simulink model "HANcoder_E407_GTSync_v5"  (R2018b)
settings: Solver=FixedStepDiscrete  StartTime=0.0  StopTime=1  FixedStep=0.01  RelTol=1e-3
PreLoadFcn:
  | librarySetup
  | eval([bdroot,'_startup']) %Calling [modelName]_startup.m
values from neighbouring files (symbols this model uses):
  basic_cycle_duration = TM_Reset_Board + COMP_duration    (= 170)    [HANcoder_E407_GTSync_v5_startup.m]
  comm_delay_estimation1 = round(comm_delay_measured*hardware_granularity/frequency_IRQ)    [HANcoder_E407_GTSync_v5_startup.m]
  comm_delay_estimation2 = round(comm_delay_measured*hardware_granularity/frequency_IRQ)    [HANcoder_E407_GTSync_v5_startup.m]
  COMM_Period = 25    [HANcoder_E407_GTSync_v5_startup.m]
  COMM_Phase1 = floor(COMM_Period/5)    [HANcoder_E407_GTSync_v5_startup.m]
  COMM_Phase2 = floor(4*COMM_Period/5)    [HANcoder_E407_GTSync_v5_startup.m]
  frequency_IRQ = 100    [HANcoder_E407_GTSync_v5_startup.m]
  HANtuneOverride = Simulink.Parameter    [HANcoder_E407_GTSync_v5_startup.m]
  idle_time_init = basic_cycle_duration*matrix_rows    (= 340)    [HANcoder_E407_GTSync_v5_startup.m]
  LED_ticks_toggle = 10000    [HANcoder_E407_GTSync_v5_startup.m]
  Master_Role = 1    [HANcoder_E407_GTSync_v5_startup.m]
  matrix_rows = 2    [HANcoder_E407_GTSync_v5_startup.m]
  MEX_Flag = 0    [HANcoder_E407_GTSync_v5_startup.m]
  Slave_Role = 2    [HANcoder_E407_GTSync_v5_startup.m]
  Sync_ID = 1    [HANcoder_E407_GTSync_v5_startup.m]
  TM_Check_Sync = TM_COMM_Sync   + COMM_duration    (= 30)    [HANcoder_E407_GTSync_v5_startup.m]
  TM_Check_TOuts = TM_Count_Vote3 + COMP_duration    (= 150)    [HANcoder_E407_GTSync_v5_startup.m]
  TM_Check_Vote1 = TM_COMM_Vote1  + COMM_duration    (= 70)    [HANcoder_E407_GTSync_v5_startup.m]
  TM_Check_Vote2 = TM_COMM_Vote2  + COMM_duration    (= 105)    [HANcoder_E407_GTSync_v5_startup.m]
  TM_Check_Vote3 = TM_COMM_Vote3  + COMM_duration    (= 140)    [HANcoder_E407_GTSync_v5_startup.m]
  TM_COMM_Sync = basic_cycle_start    (= 5)    [HANcoder_E407_GTSync_v5_startup.m]
  TM_COMM_Vote1 = TM_Vote_Dec    + COMP_duration    (= 45)    [HANcoder_E407_GTSync_v5_startup.m]
  TM_COMM_Vote2 = TM_Count_Vote1 + COMP_duration    (= 80)    [HANcoder_E407_GTSync_v5_startup.m]
  TM_COMM_Vote3 = TM_Count_Vote2 + COMP_duration    (= 115)    [HANcoder_E407_GTSync_v5_startup.m]
  TM_Count_Vote1 = TM_Check_Vote1 + COMP_duration    (= 75)    [HANcoder_E407_GTSync_v5_startup.m]
  TM_Count_Vote2 = TM_Check_Vote2 + COMP_duration    (= 110)    [HANcoder_E407_GTSync_v5_startup.m]
  TM_Count_Vote3 = TM_Check_Vote3 + COMP_duration    (= 145)    [HANcoder_E407_GTSync_v5_startup.m]
  TM_New_Master = TM_Check_TOuts + COMP_duration    (= 155)    [HANcoder_E407_GTSync_v5_startup.m]
  TM_Reset_Board = TM_Reset_Var   + COMP_duration    (= 165)    [HANcoder_E407_GTSync_v5_startup.m]
  TM_Reset_Var = TM_New_Master  + COMP_duration    (= 160)    [HANcoder_E407_GTSync_v5_startup.m]
  TM_Update_LT = TM_Check_Sync  + COMP_duration    (= 35)    [HANcoder_E407_GTSync_v5_startup.m]
  TM_Vote_Dec = TM_Update_LT   + COMP_duration    (= 40)    [HANcoder_E407_GTSync_v5_startup.m]
  Toggle_Flag = 1    [HANcoder_E407_GTSync_v5_startup.m]
  Vote1_ID = 12    [HANcoder_E407_GTSync_v5_startup.m]
  Vote2_ID = 22    [HANcoder_E407_GTSync_v5_startup.m]
  Vote3_ID = 32    [HANcoder_E407_GTSync_v5_startup.m]
undefined symbols (not defined in the file or in its folder): A0, A1, A2, A3, CON2
libraries: HANcoder_STM32_Target x25, hdlsllib x21, simulink x3, simulink_extras x1
(part 5 of 7)

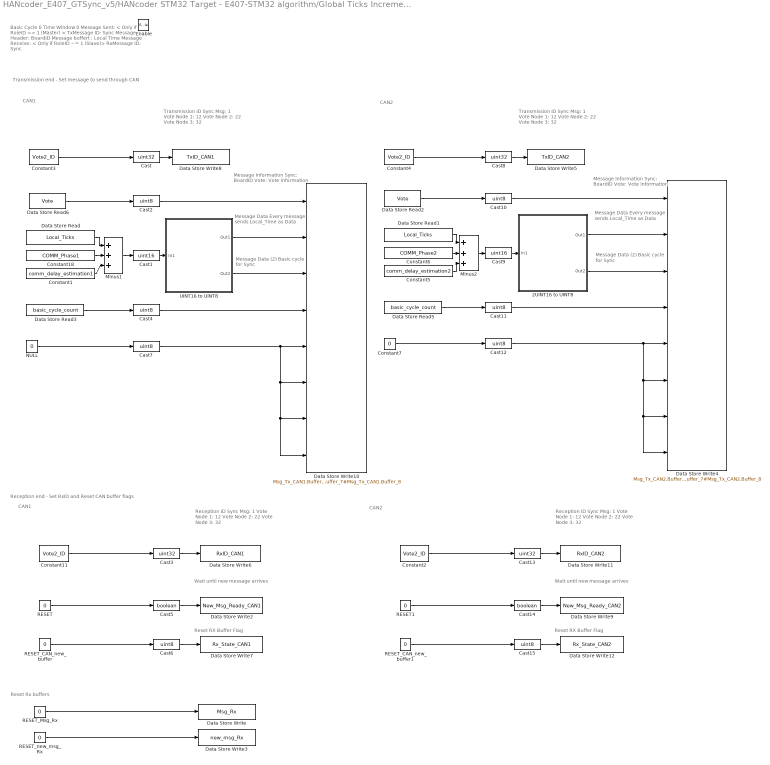
== system HANcoder_E407_GTSync_v5/HANcoder STM32 Target - E407-STM32 algorithm/Global Ticks Increment/CAN Management/Matrix Cycle Manager/COMM Task - Vote2/Vote 2 ==
  note: CAN2
  note: CAN1
  note: Transmission end - Set message to send through CAN
  note: CAN2
  note: CAN1
  note: Reception end - Set RxID and Reset CAN buffer flags
  note: Reset Rx buffers
  note: Wait until new message
      | arrives
  note: Message Data (2)
      |    Basic cycle for Sync
  note: Basic Cycle 0
      | Time Window 0
      | Message Sent: < Only if RoleID == 1 (Master) >
      | 	TxMessage ID: Sync
      | 	Message Header: BoardID
      | 	Message buffert : Local Time
      | Message Receive: < Only if RoleID ~= 1 (Slave)>
      | 	RxMessage ID: Sync
  note: Message Data
      |    Every message sends
      |    Local_Time as Data
  note: Transmission ID
      |    Sync Msg: 1
      |    Vote Node 1: 12
      |    Vote Node 2: 22
      |    Vote Node 3: 32
  note: Message Information
      |    Sync: BoardID
      |    Vote: Vote information
  note: Reception ID
      |    Sync Msg: 1
      |    Vote Node 1: 12
      |    Vote Node 2: 22
      |    Vote Node 3: 32
  note: Reset RX Buffer Flag
  note: Message Data (2)
      |    Basic cycle for Sync
  note: Message Data
      |    Every message sends
      |    Local_Time as Data
  note: Transmission ID
      |    Sync Msg: 1
      |    Vote Node 1: 12
      |    Vote Node 2: 22
      |    Vote Node 3: 32
  note: Message Information
      |    Sync: BoardID
      |    Vote: Vote information
  note: Wait until new message
      | arrives
  note: Reception ID
      |    Sync Msg: 1
      |    Vote Node 1: 12
      |    Vote Node 2: 22
      |    Vote Node 3: 32
  note: Reset RX Buffer Flag
  Enable : EnablePort
  2UINT16 to UINT8 : Subsystem
  Cast{,3,8,13} (4 alike) : DataTypeConversion  OutDataTypeStr=uint32
  Cast1 : DataTypeConversion  OutDataTypeStr=uint16
  Cast{2,4,6..7,10..12,15} (8 alike) : DataTypeConversion  OutDataTypeStr=uint8
  Cast14 : DataTypeConversion  OutDataTypeStr=boolean
  Cast5 : DataTypeConversion  OutDataTypeStr=boolean
  Cast9 : DataTypeConversion  OutDataTypeStr=uint16
  Constant1 : Constant  Value=comm_delay_estimation1
  Constant{2..4,11} (4 alike) : Constant  Value=Vote2_ID
  Constant18 : Constant  Value=COMM_Phase1
  Constant5 : Constant  Value=comm_delay_estimation2
  Constant6 : Constant  Value=COMM_Phase2
  Constant7 : Constant  Value=0  OutDataTypeStr=uint8
  Data Store Read : DataStoreRead  DataStoreName=Local_Ticks
  Data Store Read1 : DataStoreRead  DataStoreName=Local_Ticks
  Data Store Read2 : DataStoreRead  DataStoreName=Vote
  Data Store Read3 : DataStoreRead  DataStoreName=basic_cycle_count
  Data Store Read5 : DataStoreRead  DataStoreName=basic_cycle_count
  Data Store Read6 : DataStoreRead  DataStoreName=Vote
  Data Store Write : DataStoreWrite  DataStoreName=Msg_Rx
  Data Store Write10 : DataStoreWrite  DataStoreName=Msg_Tx_CAN1  DataStoreElements=Msg_Tx_CAN1.Buffer_1#Msg_Tx_CAN1.Buffer_2#Msg_Tx_CAN1.Buffer_3#Msg_Tx_CAN1.Buffer_4#Msg_Tx_CAN1.Buffer_5#Msg_Tx_CAN1.Buffer_6#Msg_Tx_CAN1.Buffer_7#Msg_Tx_CAN1.Buffer_8
  Data Store Write11 : DataStoreWrite  DataStoreName=RxID_CAN2
  Data Store Write12 : DataStoreWrite  DataStoreName=Rx_State_CAN2
  Data Store Write2 : DataStoreWrite  DataStoreName=New_Msg_Ready_CAN1
  Data Store Write3 : DataStoreWrite  DataStoreName=new_msg_Rx
  Data Store Write4 : DataStoreWrite  DataStoreName=Msg_Tx_CAN2  DataStoreElements=Msg_Tx_CAN2.Buffer_1#Msg_Tx_CAN2.Buffer_2#Msg_Tx_CAN2.Buffer_3#Msg_Tx_CAN2.Buffer_4#Msg_Tx_CAN2.Buffer_5#Msg_Tx_CAN2.Buffer_6#Msg_Tx_CAN2.Buffer_7#Msg_Tx_CAN2.Buffer_8
  Data Store Write5 : DataStoreWrite  DataStoreName=TxID_CAN2
  Data Store Write6 : DataStoreWrite  DataStoreName=RxID_CAN1
  Data Store Write7 : DataStoreWrite  DataStoreName=Rx_State_CAN1
  Data Store Write8 : DataStoreWrite  DataStoreName=TxID_CAN1
  Data Store Write9 : DataStoreWrite  DataStoreName=New_Msg_Ready_CAN2
  Minus1 : Sum  Inputs=+++
  Minus2 : Sum  Inputs=+++
  NULL : Constant  Value=0  OutDataTypeStr=uint8
  RESET : Constant  Value=0
  RESET1 : Constant  Value=0
  RESET_CAN_new_buffer : Constant  Value=0
  RESET_CAN_new_buffer1 : Constant  Value=0
  RESET_Msg_Rx : Constant  Value=0  OutDataTypeStr=Bus: demux_msg_buffer_type
  RESET_new_msg_Rx : Constant  Value=0  OutDataTypeStr=boolean
  UINT16 to UINT8 : Subsystem
  wires:
  Constant18/1 -> Minus1/2
  Minus1/1 -> Cast1/1
  Cast/1 -> Data Store Write8/1
  Data Store Read/1 -> Minus1/1
  Constant3/1 -> Cast/1
  Cast3/1 -> Data Store Write6/1
  Constant11/1 -> Cast3/1
  Cast2/1 -> Data Store Write10/1
  Cast4/1 -> Data Store Write10/4
  Data Store Read3/1 -> Cast4/1
  Data Store Read6/1 -> Cast2/1
  RESET/1 -> Cast5/1
  Cast5/1 -> Data Store Write2/1
  RESET_Msg_Rx/1 -> Data Store Write/1
  RESET_new_msg_Rx/1 -> Data Store Write3/1
  RESET_CAN_new_buffer/1 -> Cast6/1
  Cast6/1 -> Data Store Write7/1
  Constant1/1 -> Minus1/3
  Cast1/1 -> UINT16 to UINT8/1(In1)
  UINT16 to UINT8/2(Out2) -> Data Store Write10/3
  UINT16 to UINT8/1(Out1) -> Data Store Write10/2
  Cast7/1 -> Data Store Write10/8, Data Store Write10/7, Data Store Write10/6, Data Store Write10/5
  NULL/1 -> Cast7/1
  Constant7/1 -> Cast12/1
  Cast12/1 -> Data Store Write4/8, Data Store Write4/7, Data Store Write4/6, Data Store Write4/5
  2UINT16 to UINT8/1(Out1) -> Data Store Write4/2
  2UINT16 to UINT8/2(Out2) -> Data Store Write4/3
  Cast9/1 -> 2UINT16 to UINT8/1(In1)
  Constant5/1 -> Minus2/3
  Data Store Read2/1 -> Cast10/1
  Data Store Read5/1 -> Cast11/1
  Cast11/1 -> Data Store Write4/4
  Cast10/1 -> Data Store Write4/1
  Constant4/1 -> Cast8/1
  Data Store Read1/1 -> Minus2/1
  Cast8/1 -> Data Store Write5/1
  Minus2/1 -> Cast9/1
  Constant6/1 -> Minus2/2
  Cast15/1 -> Data Store Write12/1
  RESET_CAN_new_buffer1/1 -> Cast15/1
  Cast14/1 -> Data Store Write9/1
  RESET1/1 -> Cast14/1
  Constant2/1 -> Cast13/1
  Cast13/1 -> Data Store Write11/1

== system HANcoder_E407_GTSync_v5/HANcoder STM32 Target - E407-STM32 algorithm/Global Ticks Increment/CAN Management/Matrix Cycle Manager/COMM Task - Vote3/Vote 3 ==
  note: CAN2
  note: CAN1
  note: Transmission end - Set message to send through CAN
  note: CAN2
  note: CAN1
  note: Reception end - Set RxID and Reset CAN buffer flags
  note: Reset Rx buffers
  note: Wait until new message
      | arrives
  note: Message Data (2)
      |    Basic cycle for Sync
  note: Basic Cycle 0
      | Time Window 0
      | Message Sent: < Only if RoleID == 1 (Master) >
      | 	TxMessage ID: Sync
      | 	Message Header: BoardID
      | 	Message buffert : Local Time
      | Message Receive: < Only if RoleID ~= 1 (Slave)>
      | 	RxMessage ID: Sync
  note: Message Data
      |    Every message sends
      |    Local_Time as Data
  note: Transmission ID
      |    Sync Msg: 1
      |    Vote Node 1: 12
      |    Vote Node 2: 22
      |    Vote Node 3: 32
  note: Message Information
      |    Sync: BoardID
      |    Vote: Vote information
  note: Reception ID
      |    Sync Msg: 1
      |    Vote Node 1: 12
      |    Vote Node 2: 22
      |    Vote Node 3: 32
  note: Reset RX Buffer Flag
  note: Message Data (2)
      |    Basic cycle for Sync
  note: Message Data
      |    Every message sends
      |    Local_Time as Data
  note: Transmission ID
      |    Sync Msg: 1
      |    Vote Node 1: 12
      |    Vote Node 2: 22
      |    Vote Node 3: 32
  note: Message Information
      |    Sync: BoardID
      |    Vote: Vote information
  note: Wait until new message
      | arrives
  note: Reception ID
      |    Sync Msg: 1
      |    Vote Node 1: 12
      |    Vote Node 2: 22
      |    Vote Node 3: 32
  note: Reset RX Buffer Flag
  Enable : EnablePort
  2UINT16 to UINT8 : Subsystem
  Cast{,3,8,13} (4 alike) : DataTypeConversion  OutDataTypeStr=uint32
  Cast1 : DataTypeConversion  OutDataTypeStr=uint16
  Cast{2,4,6..7,10..12,15} (8 alike) : DataTypeConversion  OutDataTypeStr=uint8
  Cast14 : DataTypeConversion  OutDataTypeStr=boolean
  Cast5 : DataTypeConversion  OutDataTypeStr=boolean
  Cast9 : DataTypeConversion  OutDataTypeStr=uint16
  Constant1 : Constant  Value=comm_delay_estimation1
  Constant{2..4,11} (4 alike) : Constant  Value=Vote3_ID
  Constant18 : Constant  Value=COMM_Phase1
  Constant5 : Constant  Value=comm_delay_estimation2
  Constant6 : Constant  Value=COMM_Phase2
  Constant7 : Constant  Value=0  OutDataTypeStr=uint8
  Data Store Read : DataStoreRead  DataStoreName=Local_Ticks
  Data Store Read1 : DataStoreRead  DataStoreName=Local_Ticks
  Data Store Read2 : DataStoreRead  DataStoreName=Vote
  Data Store Read3 : DataStoreRead  DataStoreName=basic_cycle_count
  Data Store Read5 : DataStoreRead  DataStoreName=basic_cycle_count
  Data Store Read6 : DataStoreRead  DataStoreName=Vote
  Data Store Write : DataStoreWrite  DataStoreName=Msg_Rx
  Data Store Write10 : DataStoreWrite  DataStoreName=Msg_Tx_CAN1  DataStoreElements=Msg_Tx_CAN1.Buffer_1#Msg_Tx_CAN1.Buffer_2#Msg_Tx_CAN1.Buffer_3#Msg_Tx_CAN1.Buffer_4#Msg_Tx_CAN1.Buffer_5#Msg_Tx_CAN1.Buffer_6#Msg_Tx_CAN1.Buffer_7#Msg_Tx_CAN1.Buffer_8
  Data Store Write11 : DataStoreWrite  DataStoreName=RxID_CAN2
  Data Store Write12 : DataStoreWrite  DataStoreName=Rx_State_CAN2
  Data Store Write2 : DataStoreWrite  DataStoreName=New_Msg_Ready_CAN1
  Data Store Write3 : DataStoreWrite  DataStoreName=new_msg_Rx
  Data Store Write4 : DataStoreWrite  DataStoreName=Msg_Tx_CAN2  DataStoreElements=Msg_Tx_CAN2.Buffer_1#Msg_Tx_CAN2.Buffer_2#Msg_Tx_CAN2.Buffer_3#Msg_Tx_CAN2.Buffer_4#Msg_Tx_CAN2.Buffer_5#Msg_Tx_CAN2.Buffer_6#Msg_Tx_CAN2.Buffer_7#Msg_Tx_CAN2.Buffer_8
  Data Store Write5 : DataStoreWrite  DataStoreName=TxID_CAN2
  Data Store Write6 : DataStoreWrite  DataStoreName=RxID_CAN1
  Data Store Write7 : DataStoreWrite  DataStoreName=Rx_State_CAN1
  Data Store Write8 : DataStoreWrite  DataStoreName=TxID_CAN1
  Data Store Write9 : DataStoreWrite  DataStoreName=New_Msg_Ready_CAN2
  Minus1 : Sum  Inputs=+++
  Minus2 : Sum  Inputs=+++
  NULL : Constant  Value=0  OutDataTypeStr=uint8
  RESET : Constant  Value=0
  RESET1 : Constant  Value=0
  RESET_CAN_new_buffer : Constant  Value=0
  RESET_CAN_new_buffer1 : Constant  Value=0
  RESET_Msg_Rx : Constant  Value=0  OutDataTypeStr=Bus: demux_msg_buffer_type
  RESET_new_msg_Rx : Constant  Value=0  OutDataTypeStr=boolean
  UINT16 to UINT8 : Subsystem
  wires:
  Constant18/1 -> Minus1/2
  Minus1/1 -> Cast1/1
  Cast/1 -> Data Store Write8/1
  Data Store Read/1 -> Minus1/1
  Constant3/1 -> Cast/1
  Cast3/1 -> Data Store Write6/1
  Constant11/1 -> Cast3/1
  Cast2/1 -> Data Store Write10/1
  Cast4/1 -> Data Store Write10/4
  Data Store Read3/1 -> Cast4/1
  Data Store Read6/1 -> Cast2/1
  RESET/1 -> Cast5/1
  Cast5/1 -> Data Store Write2/1
  RESET_Msg_Rx/1 -> Data Store Write/1
  RESET_new_msg_Rx/1 -> Data Store Write3/1
  RESET_CAN_new_buffer/1 -> Cast6/1
  Cast6/1 -> Data Store Write7/1
  Constant1/1 -> Minus1/3
  Cast1/1 -> UINT16 to UINT8/1(In1)
  UINT16 to UINT8/2(Out2) -> Data Store Write10/3
  UINT16 to UINT8/1(Out1) -> Data Store Write10/2
  Cast7/1 -> Data Store Write10/8, Data Store Write10/7, Data Store Write10/6, Data Store Write10/5
  NULL/1 -> Cast7/1
  Constant7/1 -> Cast12/1
  Cast12/1 -> Data Store Write4/8, Data Store Write4/7, Data Store Write4/6, Data Store Write4/5
  2UINT16 to UINT8/1(Out1) -> Data Store Write4/2
  2UINT16 to UINT8/2(Out2) -> Data Store Write4/3
  Cast9/1 -> 2UINT16 to UINT8/1(In1)
  Constant5/1 -> Minus2/3
  Data Store Read2/1 -> Cast10/1
  Data Store Read5/1 -> Cast11/1
  Cast11/1 -> Data Store Write4/4
  Cast10/1 -> Data Store Write4/1
  Constant4/1 -> Cast8/1
  Data Store Read1/1 -> Minus2/1
  Cast8/1 -> Data Store Write5/1
  Minus2/1 -> Cast9/1
  Constant6/1 -> Minus2/2
  Cast15/1 -> Data Store Write12/1
  RESET_CAN_new_buffer1/1 -> Cast15/1
  Cast14/1 -> Data Store Write9/1
  RESET1/1 -> Cast14/1
  Constant2/1 -> Cast13/1
  Cast13/1 -> Data Store Write11/1

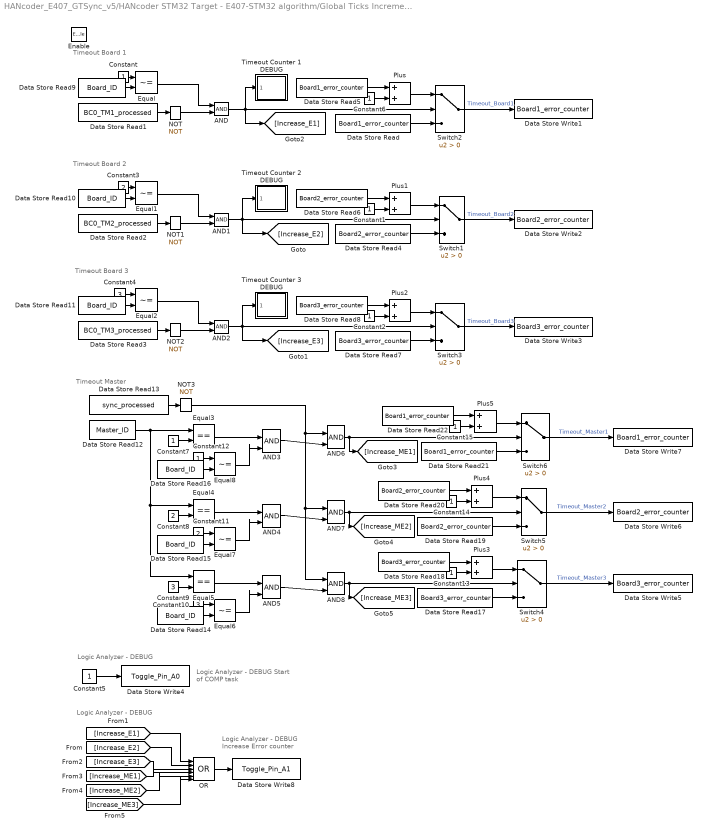
== system HANcoder_E407_GTSync_v5/HANcoder STM32 Target - E407-STM32 algorithm/Global Ticks Increment/CAN Management/Matrix Cycle Manager/COMP Task - Check Timeouts/Timeout and Board error counter ==
  note: Logic Analyzer - DEBUG
  note: Timeout Master
  note: Timeout Board 2
  note: Timeout Board 3
  note: Timeout Board 1
  note: Logic Analyzer - DEBUG
      | Start of COMP task
  note: Logic Analyzer - DEBUG
  note: Logic Analyzer - DEBUG
      | Increase Error counter
  Enable : EnablePort  PropagateVarSize=During execution
  AND{,1..8} (9 alike) : Logic  IconShape=distinctive  AllPortsSameDT=off  OutDataTypeStr=boolean
  Constant{,1..2,6..7,12..15} (9 alike) : Constant
  Constant10 : Constant  Value=3
  Constant11 : Constant  Value=2
  Constant3 : Constant  Value=2
  Constant4 : Constant  Value=3
  Constant5 : Constant  OutDataTypeStr=boolean
  Constant8 : Constant  Value=2
  Constant9 : Constant  Value=3
  Data Store Read{,5,21..22} (4 alike) : DataStoreRead  DataStoreName=Board1_error_counter
  Data Store Read1 : DataStoreRead  DataStoreName=BC0_TM1_processed
  Data Store Read{9..11,14..16} (6 alike) : DataStoreRead  DataStoreName=Board_ID
  Data Store Read12 : DataStoreRead  DataStoreName=Master_ID
  Data Store Read13 : DataStoreRead  DataStoreName=sync_processed
  Data Store Read{7..8,17..18} (4 alike) : DataStoreRead  DataStoreName=Board3_error_counter
  Data Store Read{4,6,19..20} (4 alike) : DataStoreRead  DataStoreName=Board2_error_counter
  Data Store Read2 : DataStoreRead  DataStoreName=BC0_TM2_processed
  Data Store Read3 : DataStoreRead  DataStoreName=BC0_TM3_processed
  Data Store Write1 : DataStoreWrite  DataStoreName=Board1_error_counter
  Data Store Write2 : DataStoreWrite  DataStoreName=Board2_error_counter
  Data Store Write3 : DataStoreWrite  DataStoreName=Board3_error_counter
  Data Store Write4 : DataStoreWrite  DataStoreName=Toggle_Pin_A0
  Data Store Write5 : DataStoreWrite  DataStoreName=Board3_error_counter
  Data Store Write6 : DataStoreWrite  DataStoreName=Board2_error_counter
  Data Store Write7 : DataStoreWrite  DataStoreName=Board1_error_counter
  Data Store Write8 : DataStoreWrite  DataStoreName=Toggle_Pin_A1
  Equal{,1..2,6..8} (6 alike) : RelationalOperator  Operator=~=  OutDataTypeStr=boolean  RndMeth=Simplest
  Equal3 : RelationalOperator  Operator===  OutDataTypeStr=boolean  RndMeth=Simplest
  Equal4 : RelationalOperator  Operator===  OutDataTypeStr=boolean  RndMeth=Simplest
  Equal5 : RelationalOperator  Operator===  OutDataTypeStr=boolean  RndMeth=Simplest
  NOT{,1..3} (4 alike) : Logic  Operator=NOT  IconShape=distinctive  AllPortsSameDT=off  OutDataTypeStr=boolean
  OR : Logic  Operator=OR  Inputs=6  IconShape=distinctive  AllPortsSameDT=off  OutDataTypeStr=boolean
  Plus{,1..5} (6 alike) : Sum
  Switch{1..6} (6 alike) : Switch  Criteria=u2 > Threshold
  Timeout Counter 1 DEBUG : Subsystem
  Timeout Counter 2 DEBUG : Subsystem
  Timeout Counter 3 DEBUG : Subsystem
  wires:
  Constant6/1 -> Plus/2
  Plus/1 -> Switch2/1
  Plus2/1 -> Switch3/1
  Plus1/1 -> Switch1/1
  NOT/1 -> AND/2
  Data Store Read7/1 -> Switch3/3
  NOT2/1 -> AND2/2
  Data Store Read2/1 -> NOT1/1
  Equal2/1 -> AND2/1
  Equal1/1 -> AND1/1
  Data Store Read6/1 -> Plus1/1
  Data Store Read8/1 -> Plus2/1
  Data Store Read3/1 -> NOT2/1
  Switch3/1 -> Data Store Write3/1  "Timeout_Board3"
  Switch2/1 -> Data Store Write1/1  "Timeout_Board1"
  Constant1/1 -> Plus1/2
  Data Store Read5/1 -> Plus/1
  Data Store Read1/1 -> NOT/1
  Data Store Read9/1 -> Equal/2
  NOT1/1 -> AND1/2
  AND2/1 -> [Increase_E3], Timeout Counter 3 DEBUG/1(Timeout), Switch3/2
  Constant2/1 -> Plus2/2
  Data Store Read/1 -> Switch2/3
  Constant4/1 -> Equal2/1
  Data Store Read4/1 -> Switch1/3
  Data Store Read10/1 -> Equal1/2
  Constant/1 -> Equal/1
  Switch1/1 -> Data Store Write2/1  "Timeout_Board2"
  Data Store Read11/1 -> Equal2/2
  Equal/1 -> AND/1
  Constant3/1 -> Equal1/1
  Constant5/1 -> Data Store Write4/1
  Data Store Read13/1 -> NOT3/1
  NOT3/1 -> AND8/1, AND7/1, AND6/1
  Data Store Read12/1 -> Equal3/1, Equal4/1, Equal5/1
  Constant7/1 -> Equal3/2
  Constant8/1 -> Equal4/2
  Constant9/1 -> Equal5/2
  Data Store Read14/1 -> Equal6/2
  Constant10/1 -> Equal6/1
  Constant11/1 -> Equal7/1
  Data Store Read15/1 -> Equal7/2
  Data Store Read16/1 -> Equal8/2
  Constant12/1 -> Equal8/1
  Equal3/1 -> AND3/1
  Equal8/1 -> AND3/2
  Equal4/1 -> AND4/1
  Equal7/1 -> AND4/2
  Equal5/1 -> AND5/1
  Equal6/1 -> AND5/2
  AND3/1 -> AND6/2
  AND5/1 -> AND8/2
  AND4/1 -> AND7/2
  Constant13/1 -> Plus3/2
  AND8/1 -> Switch4/2, [Increase_ME3]
  Switch4/1 -> Data Store Write5/1  "Timeout_Master3"
  Data Store Read18/1 -> Plus3/1
  Data Store Read17/1 -> Switch4/3
  Plus3/1 -> Switch4/1
  Switch5/1 -> Data Store Write6/1  "Timeout_Master2"
  Data Store Read19/1 -> Switch5/3
  AND7/1 -> [Increase_ME2], Switch5/2
  Constant14/1 -> Plus4/2
  Data Store Read20/1 -> Plus4/1
  Plus4/1 -> Switch5/1
  AND6/1 -> [Increase_ME1], Switch6/2
  Data Store Read21/1 -> Switch6/3
  Data Store Read22/1 -> Plus5/1
  Switch6/1 -> Data Store Write7/1  "Timeout_Master1"
  Plus5/1 -> Switch6/1
  Constant15/1 -> Plus5/2
  AND1/1 -> [Increase_E2], Timeout Counter 2 DEBUG/1(Timeout), Switch1/2
  AND/1 -> [Increase_E1], Timeout Counter 1 DEBUG/1(Timeout), Switch2/2
  [Increase_E1] -> OR/1
  [Increase_E2] -> OR/2
  [Increase_E3] -> OR/3
  OR/1 -> Data Store Write8/1
  [Increase_ME1] -> OR/4
  [Increase_ME3] -> OR/6
  [Increase_ME2] -> OR/5

== system HANcoder_E407_GTSync_v5/HANcoder STM32 Target - E407-STM32 algorithm/Global Ticks Increment/CAN Management/Matrix Cycle Manager/COMP Task - New Master/New Master ==
  note: Post voting process
  note: Logic Analyzer - DEBUG
      | Start of COMP task
  note: Logic Analyzer - DEBUG
  Enable : EnablePort  PropagateVarSize=During execution
  Constant10 : Constant  Value=Slave_Role
  Constant3 : Constant  OutDataTypeStr=boolean
  Constant9 : Constant  Value=Master_Role
  Data Store Read : DataStoreRead  DataStoreName=Master_ID
  Data Store Read27 : DataStoreRead  DataStoreName=Board_ID
  Data Store Write : DataStoreWrite  DataStoreName=Reset_Board
  Data Store Write1 : DataStoreWrite  DataStoreName=New_Master
  Data Store Write13 : DataStoreWrite  DataStoreName=Master_ID
  Data Store Write15 : DataStoreWrite  DataStoreName=Role_ID
  Data Store Write3 : DataStoreWrite  DataStoreName=Toggle_Pin_A0
  Equal : RelationalOperator  Operator=~=  OutDataTypeStr=boolean  RndMeth=Simplest
  Equal6 : RelationalOperator  Operator===  OutDataTypeStr=boolean  RndMeth=Simplest
  Switch16 : Switch  Criteria=u2 > Threshold
  Votes recount to choose Master : Subsystem
  wires:
  Equal6/1 -> Switch16/2
  Data Store Read27/1 -> Equal6/2
  Switch16/1 -> Data Store Write15/1  "Role_ID_s"
  Constant9/1 -> Switch16/1
  Constant10/1 -> Switch16/3
  Data Store Read/1 -> Equal/1
  Equal/1 -> Data Store Write1/1
  Votes recount to choose Master/1(Master_ID_s) -> Equal6/1, Equal/2, Data Store Write13/1
  Votes recount to choose Master/2(Reset Board) -> Data Store Write/1
  Constant3/1 -> Data Store Write3/1

== system HANcoder_E407_GTSync_v5/HANcoder STM32 Target - E407-STM32 algorithm/Global Ticks Increment/CAN Management/Matrix Cycle Manager/COMP Task - Reset Board/RESET Board - Return to initialization ==
  note: Role reset
  note: CAN Rx preparation for sync
  note: Reset board state
  note: Logic Analyzer - DEBUG
      | Start of COMP task
  note: Logic Analyzer - DEBUG
  Enable : EnablePort
  Cast : DataTypeConversion  OutDataTypeStr=boolean
  Cast6 : DataTypeConversion  OutDataTypeStr=uint8
  Constant : Constant  Value=0
  Constant1 : Constant  Value=Sync_ID  OutDataTypeStr=uint32
  Constant3 : Constant  OutDataTypeStr=boolean
  Data Store Write : DataStoreWrite  DataStoreName=Reset_Board
  Data Store Write1 : DataStoreWrite  DataStoreName=New_Msg_Ready_CAN1
  Data Store Write10 : DataStoreWrite  DataStoreName=New_Msg_Ready_CAN2
  Data Store Write2 : DataStoreWrite  DataStoreName=Initialization_flag
  Data Store Write3 : DataStoreWrite  DataStoreName=RxID_CAN1
  Data Store Write4 : DataStoreWrite  DataStoreName=Role_ID
  Data Store Write5 : DataStoreWrite  DataStoreName=Master_ID
  Data Store Write6 : DataStoreWrite  DataStoreName=Rx_State_CAN1
  Data Store Write7 : DataStoreWrite  DataStoreName=Toggle_Pin_A0
  Data Store Write8 : DataStoreWrite  DataStoreName=RxID_CAN2
  Data Store Write9 : DataStoreWrite  DataStoreName=Rx_State_CAN2
  NOT : Logic  Operator=NOT  IconShape=distinctive  AllPortsSameDT=off  OutDataTypeStr=boolean
  wires:
  Constant/1 -> Data Store Write5/1, Data Store Write4/1, Cast6/1, Cast/1
  Cast/1 -> Data Store Write10/1, Data Store Write1/1, NOT/1, Data Store Write/1
  NOT/1 -> Data Store Write2/1
  Constant1/1 -> Data Store Write8/1, Data Store Write3/1
  Cast6/1 -> Data Store Write9/1, Data Store Write6/1
  Constant3/1 -> Data Store Write7/1

== system HANcoder_E407_GTSync_v5/HANcoder STM32 Target - E407-STM32 algorithm/Global Ticks Increment/CAN Management/Matrix Cycle Manager/COMP Task - Reset Variables BC0/Reset variables ==
  note: Reset variables
  note: Logic Analyzer - DEBUG
      | Start of COMP task
  note: Logic Analyzer - DEBUG
  Enable : EnablePort
  Cast : DataTypeConversion  OutDataTypeStr=boolean
  Constant : Constant  Value=0
  Constant3 : Constant  OutDataTypeStr=boolean
  Data Store Write1 : DataStoreWrite  DataStoreName=sync_processed
  Data Store Write16 : DataStoreWrite  DataStoreName=votes  DataStoreElements=votes.First_Board#votes.Second_Board#votes.Third_Board
  Data Store Write2 : DataStoreWrite  DataStoreName=BC0_TM1_processed
  Data Store Write3 : DataStoreWrite  DataStoreName=BC0_TM2_processed
  Data Store Write4 : DataStoreWrite  DataStoreName=BC0_TM3_processed
  Data Store Write5 : DataStoreWrite  DataStoreName=Toggle_Pin_A0
  wires:
  Constant/1 -> Data Store Write16/1, Cast/1, Data Store Write16/3, Data Store Write16/2
  Cast/1 -> Data Store Write4/1, Data Store Write3/1, Data Store Write2/1, Data Store Write1/1
  Constant3/1 -> Data Store Write5/1

== system HANcoder_E407_GTSync_v5/HANcoder STM32 Target - E407-STM32 algorithm/Global Ticks Increment/CAN Management/Matrix Cycle Manager/COMP Task - Reset Variables BC1/Reset Variables ==
  note: Reset variables
  note: Logic Analyzer - DEBUG
      | Start of COMP task
  note: Logic Analyzer - DEBUG
  Enable : EnablePort
  Cast : DataTypeConversion  OutDataTypeStr=boolean
  Constant : Constant  Value=0
  Constant3 : Constant  OutDataTypeStr=boolean
  Data Store Write1 : DataStoreWrite  DataStoreName=sync_processed
  Data Store Write3 : DataStoreWrite  DataStoreName=Toggle_Pin_A0
  wires:
  Constant/1 -> Cast/1
  Cast/1 -> Data Store Write1/1
  Constant3/1 -> Data Store Write3/1

== system HANcoder_E407_GTSync_v5/HANcoder STM32 Target - E407-STM32 algorithm/Global Ticks Increment/CAN Management/Matrix Cycle Manager/COMP Task - Rx_Sync_Check/Process_Messages ==
  note: Desync CAN2
      | expected RX - Actual RX
  note: Desync CAN1
      | expected RX - Actual RX
  new_CAN1_msg : Inport
  new_CAN2_msg : Inport  Port=2
  Rx_msg_CAN1 : Inport  Port=3  OutDataTypeStr=Bus: msg_buffer_type
  Rx_Msg_CAN2 : Inport  Port=4  OutDataTypeStr=Bus: msg_buffer_type
  expected_msg_header : Inport  Port=5
  expected_local_time : Inport  Port=6
  expected_basic_cycle : Inport  Port=7
  Enable : EnablePort
  Bus Selector : BusSelector  OutputSignals=Buffer_1,signal2,Buffer_4
  Constant : Constant  Value=COMM_Phase1
  Constant1 : Constant  Value=COMM_Phase2
  Data Store Read : DataStoreRead  DataStoreName=Msg_Rx_Ticks_CAN1
  Data Store Read1 : DataStoreRead  DataStoreName=Msg_Rx_Ticks_CAN2
  Data Store Write : DataStoreWrite  DataStoreName=Msg_Rx  DataStoreElements=Msg_Rx.Msg_Header#Msg_Rx.Local_Time#Msg_Rx.Basic_Cycle
  Data Store Write1 : DataStoreWrite  DataStoreName=Desync_Ticks
  Data Store Write2 : DataStoreWrite  DataStoreName=new_msg_Rx
  Demux message CAN1 and check coherence : Subsystem
  Demux message CAN2 and check coherence : Subsystem
  Minus : Sum  Inputs=+-
  Minus1 : Sum  Inputs=+-
  OR : Logic  Operator=OR  IconShape=distinctive  AllPortsSameDT=off  OutDataTypeStr=boolean
  Sum : Sum  Inputs=+++
  Sum1 : Sum  Inputs=+++
  Switch : Switch  Criteria=u2 > Threshold
  Switch1 : Switch  Criteria=u2 > Threshold
  delay_estimation_1 : Constant  Value=comm_delay_estimation1
  delay_estimation_2 : Constant  Value=comm_delay_estimation2
  wires:
  new_CAN1_msg/1 -> Demux message CAN1 and check coherence/Enable, Switch1/2
  new_CAN2_msg/1 -> Demux message CAN2 and check coherence/Enable
  Rx_msg_CAN1/1 -> Demux message CAN1 and check coherence/1(CAN1_Rx_msg)
  Rx_Msg_CAN2/1 -> Demux message CAN2 and check coherence/1(CAN2_Rx_msg)
  Demux message CAN1 and check coherence/2(CAN1_msg_coherent) -> Switch/2, OR/1
  Demux message CAN1 and check coherence/1(CAN1_msg) -> Switch/1
  Demux message CAN2 and check coherence/1(CAN2_msg_coherent) -> OR/2
  Demux message CAN2 and check coherence/2(CAN2_msg) -> Switch/3
  OR/1 -> Data Store Write2/1  "new_msg_Rx_Sync_s"
  Switch/1 -> Bus Selector/1
  expected_local_time/1 -> Sum1/2, Sum/2
  expected_basic_cycle/1 -> Demux message CAN1 and check coherence/4(expected_basic_cycle), Demux message CAN2 and check coherence/4(expected_basic_cycle)
  Sum/1 -> [expected_LT_CAN1], Demux message CAN1 and check coherence/3(expected_local_time)
  Sum1/1 -> [expected_LT_CAN2], Demux message CAN2 and check coherence/3(expected_local_time)
  Minus1/1 -> Switch1/1
  Minus/1 -> Switch1/3
  Switch1/1 -> Data Store Write1/1  "Desync_Sync_bc0_s"
  Bus Selector/1 -> Data Store Write/1  "<Buffer_1>"
  Bus Selector/2 -> Data Store Write/2  "<signal2>"
  Bus Selector/3 -> Data Store Write/3  "<Buffer_4>"
  Constant/1 -> Sum/1
  delay_estimation_1/1 -> Sum/3
  Constant1/1 -> Sum1/1
  expected_msg_header/1 -> Demux message CAN1 and check coherence/2(expected_msg_header), Demux message CAN2 and check coherence/2(expected_msg_header)
  delay_estimation_2/1 -> Sum1/3
  Data Store Read1/1 -> Minus/2
  [expected_LT_CAN2] -> Minus/1
  [expected_LT_CAN1] -> Minus1/1
  Data Store Read/1 -> Minus1/2

== system HANcoder_E407_GTSync_v5/HANcoder STM32 Target - E407-STM32 algorithm/Global Ticks Increment/CAN Management/Matrix Cycle Manager/COMP Task - Rx_Sync_Check - bc1/Process_Messages ==
  note: Desync CAN2
      | expected RX - Actual RX
  note: Desync CAN1
      | expected RX - Actual RX
  new_CAN1_msg : Inport
  new_CAN2_msg : Inport  Port=2
  Rx_msg_CAN1 : Inport  Port=3  OutDataTypeStr=Bus: msg_buffer_type
  Rx_Msg_CAN2 : Inport  Port=4  OutDataTypeStr=Bus: msg_buffer_type
  expected_msg_header : Inport  Port=5
  expected_local_time : Inport  Port=6
  expected_basic_cycle : Inport  Port=7
  Enable : EnablePort
  Bus Selector : BusSelector  OutputSignals=Buffer_1,signal2,Buffer_4
  Constant : Constant  Value=COMM_Phase1
  Constant1 : Constant  Value=COMM_Phase2
  Data Store Read : DataStoreRead  DataStoreName=Msg_Rx_Ticks_CAN1
  Data Store Read1 : DataStoreRead  DataStoreName=Msg_Rx_Ticks_CAN2
  Data Store Write : DataStoreWrite  DataStoreName=Msg_Rx  DataStoreElements=Msg_Rx.Msg_Header#Msg_Rx.Local_Time#Msg_Rx.Basic_Cycle
  Data Store Write1 : DataStoreWrite  DataStoreName=new_msg_Rx
  Data Store Write2 : DataStoreWrite  DataStoreName=Desync_Ticks
  Demux message CAN1 and check coherence : Subsystem
  Demux message CAN2 and check coherence : Subsystem
  Minus : Sum  Inputs=+-
  Minus1 : Sum  Inputs=+-
  OR : Logic  Operator=OR  IconShape=distinctive  AllPortsSameDT=off  OutDataTypeStr=boolean
  Sum : Sum  Inputs=+++
  Sum1 : Sum  Inputs=+++
  Switch : Switch  Criteria=u2 > Threshold
  Switch1 : Switch  Criteria=u2 > Threshold
  delay_estimation_1 : Constant  Value=comm_delay_estimation1
  delay_estimation_2 : Constant  Value=comm_delay_estimation2
  wires:
  new_CAN2_msg/1 -> Demux message CAN2 and check coherence/Enable
  Rx_msg_CAN1/1 -> Demux message CAN1 and check coherence/1(CAN1_Rx_msg)
  Rx_Msg_CAN2/1 -> Demux message CAN2 and check coherence/1(CAN2_Rx_msg)
  Demux message CAN1 and check coherence/2(CAN1_msg_coherent) -> Switch/2, OR/1
  Demux message CAN1 and check coherence/1(CAN1_msg) -> Switch/1
  Demux message CAN2 and check coherence/1(CAN2_msg_coherent) -> OR/2
  Demux message CAN2 and check coherence/2(CAN2_msg) -> Switch/3
  OR/1 -> Data Store Write1/1
  Switch/1 -> Bus Selector/1
  expected_msg_header/1 -> Demux message CAN1 and check coherence/2(expected_msg_header), Demux message CAN2 and check coherence/2(expected_msg_header)
  expected_basic_cycle/1 -> Demux message CAN1 and check coherence/4(expected_basic_cycle), Demux message CAN2 and check coherence/4(expected_basic_cycle)
  Bus Selector/1 -> Data Store Write/1  "<Buffer_1>"
  Bus Selector/2 -> Data Store Write/2  "<signal2>"
  Bus Selector/3 -> Data Store Write/3  "<Buffer_4>"
  Data Store Read1/1 -> Minus/2
  Switch1/1 -> Data Store Write2/1  "Desync_Sync_bc1_s"
  new_CAN1_msg/1 -> Switch1/2, Demux message CAN1 and check coherence/Enable
  [expected_LT_CAN2] -> Minus/1
  Minus/1 -> Switch1/3
  Data Store Read/1 -> Minus1/2
  [expected_LT_CAN1] -> Minus1/1
  Minus1/1 -> Switch1/1
  delay_estimation_1/1 -> Sum/3
  Sum/1 -> [expected_LT_CAN1], Demux message CAN1 and check coherence/3(expected_local_time)
  Constant/1 -> Sum/1
  delay_estimation_2/1 -> Sum1/3
  expected_local_time/1 -> Sum1/2, Sum/2
  Sum1/1 -> [expected_LT_CAN2], Demux message CAN2 and check coherence/3(expected_local_time)
  Constant1/1 -> Sum1/1

== system HANcoder_E407_GTSync_v5/HANcoder STM32 Target - E407-STM32 algorithm/Global Ticks Increment/CAN Management/Matrix Cycle Manager/COMP Task - Rx_Vote1_Check/Process_Messages1 ==
  note: Desync CAN2
      | expected RX - Actual RX
  note: Desync CAN1
      | expected RX - Actual RX
  new_CAN1_msg : Inport
  new_CAN2_msg : Inport  Port=2
  Rx_msg_CAN1 : Inport  Port=3  OutDataTypeStr=Bus: msg_buffer_type
  Rx_Msg_CAN2 : Inport  Port=4  OutDataTypeStr=Bus: msg_buffer_type
  expected_local_time : Inport  Port=5
  expected_basic_cycle : Inport  Port=6
  Enable : EnablePort
  Bus Selector : BusSelector  OutputSignals=Buffer_1,signal2,Buffer_4
  Constant : Constant  Value=COMM_Phase1
  Constant1 : Constant  Value=COMM_Phase2
  Data Store Read : DataStoreRead  DataStoreName=Msg_Rx_Ticks_CAN1
  Data Store Read1 : DataStoreRead  DataStoreName=Msg_Rx_Ticks_CAN2
  Data Store Write : DataStoreWrite  DataStoreName=Msg_Rx  DataStoreElements=Msg_Rx.Msg_Header#Msg_Rx.Local_Time#Msg_Rx.Basic_Cycle
  Data Store Write1 : DataStoreWrite  DataStoreName=new_msg_Rx
  Data Store Write2 : DataStoreWrite  DataStoreName=Desync_Ticks
  Demux message CAN1 and check coherence : Subsystem
  Demux message CAN2 and check coherence : Subsystem
  Minus : Sum  Inputs=+-
  Minus1 : Sum  Inputs=+-
  OR : Logic  Operator=OR  IconShape=distinctive  AllPortsSameDT=off  OutDataTypeStr=boolean
  Sum : Sum  Inputs=+++
  Sum1 : Sum  Inputs=+++
  Switch : Switch  Criteria=u2 > Threshold
  Switch1 : Switch  Criteria=u2 > Threshold
  delay_estimation_1 : Constant  Value=comm_delay_estimation1
  delay_estimation_2 : Constant  Value=comm_delay_estimation2
  wires:
  new_CAN2_msg/1 -> Demux message CAN2 and check coherence/Enable
  Rx_msg_CAN1/1 -> Demux message CAN1 and check coherence/1(CAN1_Rx_msg)
  Rx_Msg_CAN2/1 -> Demux message CAN2 and check coherence/1(CAN2_Rx_msg)
  Demux message CAN1 and check coherence/2(CAN1_msg_coherent) -> Switch/2, OR/1
  Demux message CAN1 and check coherence/1(CAN1_msg) -> Switch/1
  Demux message CAN2 and check coherence/1(CAN2_msg_coherent) -> OR/2
  Demux message CAN2 and check coherence/2(CAN2_msg) -> Switch/3
  OR/1 -> Data Store Write1/1  "new_msg_Rx_Vote1_s"
  Switch/1 -> Bus Selector/1
  expected_basic_cycle/1 -> Demux message CAN1 and check coherence/3(expected_basic_cycle), Demux message CAN2 and check coherence/3(expected_basic_cycle)
  Sum/1 -> [expected_LT_CAN1], Demux message CAN1 and check coherence/2(expected_local_time)
  Bus Selector/1 -> Data Store Write/1  "<Buffer_1>"
  Bus Selector/2 -> Data Store Write/2  "<signal2>"
  Bus Selector/3 -> Data Store Write/3  "<Buffer_4>"
  Constant/1 -> Sum/1
  delay_estimation_1/1 -> Sum/3
  Constant1/1 -> Sum1/1
  expected_local_time/1 -> Sum1/2, Sum/2
  delay_estimation_2/1 -> Sum1/3
  Sum1/1 -> [expected_LT_CAN2], Demux message CAN2 and check coherence/2(expected_local_time)
  Data Store Read1/1 -> Minus/2
  Switch1/1 -> Data Store Write2/1  "Desync_Vote1_s"
  new_CAN1_msg/1 -> Switch1/2, Demux message CAN1 and check coherence/Enable
  [expected_LT_CAN2] -> Minus/1
  Minus/1 -> Switch1/3
  Data Store Read/1 -> Minus1/2
  [expected_LT_CAN1] -> Minus1/1
  Minus1/1 -> Switch1/1

== system HANcoder_E407_GTSync_v5/HANcoder STM32 Target - E407-STM32 algorithm/Global Ticks Increment/CAN Management/Matrix Cycle Manager/COMP Task - Rx_Vote2_Check/Process_Messages1 ==
  note: Desync CAN2
      | expected RX - Actual RX
  note: Desync CAN1
      | expected RX - Actual RX
  new_CAN1_msg : Inport
  new_CAN2_msg : Inport  Port=2
  Rx_msg_CAN1 : Inport  Port=3  OutDataTypeStr=Bus: msg_buffer_type
  Rx_Msg_CAN2 : Inport  Port=4  OutDataTypeStr=Bus: msg_buffer_type
  expected_local_time : Inport  Port=5
  expected_basic_cycle : Inport  Port=6
  Enable : EnablePort
  Bus Selector : BusSelector  OutputSignals=Buffer_1,signal2,Buffer_4
  Constant : Constant  Value=COMM_Phase1
  Constant1 : Constant  Value=COMM_Phase2
  Data Store Read : DataStoreRead  DataStoreName=Msg_Rx_Ticks_CAN1
  Data Store Read1 : DataStoreRead  DataStoreName=Msg_Rx_Ticks_CAN2
  Data Store Write : DataStoreWrite  DataStoreName=Msg_Rx  DataStoreElements=Msg_Rx.Msg_Header#Msg_Rx.Local_Time#Msg_Rx.Basic_Cycle
  Data Store Write1 : DataStoreWrite  DataStoreName=new_msg_Rx
  Data Store Write2 : DataStoreWrite  DataStoreName=Desync_Ticks
  Demux message CAN1 and check coherence : Subsystem
  Demux message CAN2 and check coherence : Subsystem
  Minus : Sum  Inputs=+-
  Minus1 : Sum  Inputs=+-
  OR : Logic  Operator=OR  IconShape=distinctive  AllPortsSameDT=off  OutDataTypeStr=boolean
  Sum : Sum  Inputs=+++
  Sum1 : Sum  Inputs=+++
  Switch : Switch  Criteria=u2 > Threshold
  Switch1 : Switch  Criteria=u2 > Threshold
  delay_estimation_1 : Constant  Value=comm_delay_estimation1
  delay_estimation_2 : Constant  Value=comm_delay_estimation2
  wires:
  new_CAN2_msg/1 -> Demux message CAN2 and check coherence/Enable
  Rx_msg_CAN1/1 -> Demux message CAN1 and check coherence/1(CAN1_Rx_msg)
  Rx_Msg_CAN2/1 -> Demux message CAN2 and check coherence/1(CAN2_Rx_msg)
  Demux message CAN1 and check coherence/2(CAN1_msg_coherent) -> Switch/2, OR/1
  Demux message CAN1 and check coherence/1(CAN1_msg) -> Switch/1
  Demux message CAN2 and check coherence/1(CAN2_msg_coherent) -> OR/2
  Demux message CAN2 and check coherence/2(CAN2_msg) -> Switch/3
  OR/1 -> Data Store Write1/1  "new_msg_Rx_Vote2_s"
  Switch/1 -> Bus Selector/1
  expected_basic_cycle/1 -> Demux message CAN1 and check coherence/3(expected_basic_cycle), Demux message CAN2 and check coherence/3(expected_basic_cycle)
  Sum/1 -> [expected_LT_CAN1], Demux message CAN1 and check coherence/2(expected_local_time)
  Sum1/1 -> [expected_LT_CAN2], Demux message CAN2 and check coherence/2(expected_local_time)
  Bus Selector/1 -> Data Store Write/1  "<Buffer_1>"
  Bus Selector/2 -> Data Store Write/2  "<signal2>"
  Bus Selector/3 -> Data Store Write/3  "<Buffer_4>"
  Constant/1 -> Sum/1
  delay_estimation_1/1 -> Sum/3
  Constant1/1 -> Sum1/1
  expected_local_time/1 -> Sum1/2, Sum/2
  delay_estimation_2/1 -> Sum1/3
  Data Store Read1/1 -> Minus/2
  Switch1/1 -> Data Store Write2/1  "Desync_Vote2_s"
  new_CAN1_msg/1 -> Switch1/2, Demux message CAN1 and check coherence/Enable
  [expected_LT_CAN2] -> Minus/1
  Minus/1 -> Switch1/3
  Data Store Read/1 -> Minus1/2
  [expected_LT_CAN1] -> Minus1/1
  Minus1/1 -> Switch1/1

== system HANcoder_E407_GTSync_v5/HANcoder STM32 Target - E407-STM32 algorithm/Global Ticks Increment/CAN Management/Matrix Cycle Manager/COMP Task - Rx_Vote3_Check/Process_Messages1 ==
  note: Desync CAN2
      | expected RX - Actual RX
  note: Desync CAN1
      | expected RX - Actual RX
  new_CAN1_msg : Inport
  new_CAN2_msg : Inport  Port=2
  Rx_msg_CAN1 : Inport  Port=3  OutDataTypeStr=Bus: msg_buffer_type
  Rx_Msg_CAN2 : Inport  Port=4  OutDataTypeStr=Bus: msg_buffer_type
  expected_local_time : Inport  Port=5
  expected_basic_cycle : Inport  Port=6
  Enable : EnablePort
  Bus Selector : BusSelector  OutputSignals=Buffer_1,signal2,Buffer_4
  Constant : Constant  Value=COMM_Phase1
  Constant1 : Constant  Value=COMM_Phase2
  Data Store Read : DataStoreRead  DataStoreName=Msg_Rx_Ticks_CAN1
  Data Store Read1 : DataStoreRead  DataStoreName=Msg_Rx_Ticks_CAN2
  Data Store Write : DataStoreWrite  DataStoreName=Msg_Rx  DataStoreElements=Msg_Rx.Msg_Header#Msg_Rx.Local_Time#Msg_Rx.Basic_Cycle
  Data Store Write1 : DataStoreWrite  DataStoreName=new_msg_Rx
  Data Store Write2 : DataStoreWrite  DataStoreName=Desync_Ticks
  Demux message CAN1 and check coherence : Subsystem
  Demux message CAN2 and check coherence : Subsystem
  Minus : Sum  Inputs=+-
  Minus1 : Sum  Inputs=+-
  OR : Logic  Operator=OR  IconShape=distinctive  AllPortsSameDT=off  OutDataTypeStr=boolean
  Sum : Sum  Inputs=+++
  Sum1 : Sum  Inputs=+++
  Switch : Switch  Criteria=u2 > Threshold
  Switch1 : Switch  Criteria=u2 > Threshold
  delay_estimation_1 : Constant  Value=comm_delay_estimation1
  delay_estimation_2 : Constant  Value=comm_delay_estimation2
  wires:
  new_CAN2_msg/1 -> Demux message CAN2 and check coherence/Enable
  Rx_msg_CAN1/1 -> Demux message CAN1 and check coherence/1(CAN1_Rx_msg)
  Rx_Msg_CAN2/1 -> Demux message CAN2 and check coherence/1(CAN2_Rx_msg)
  Demux message CAN1 and check coherence/2(CAN1_msg_coherent) -> Switch/2, OR/1
  Demux message CAN1 and check coherence/1(CAN1_msg) -> Switch/1
  Demux message CAN2 and check coherence/1(CAN2_msg_coherent) -> OR/2
  Demux message CAN2 and check coherence/2(CAN2_msg) -> Switch/3
  OR/1 -> Data Store Write1/1  "new_msg_Rx_Vote3_s"
  Switch/1 -> Bus Selector/1
  expected_basic_cycle/1 -> Demux message CAN1 and check coherence/3(expected_basic_cycle), Demux message CAN2 and check coherence/3(expected_basic_cycle)
  Bus Selector/1 -> Data Store Write/1  "<Buffer_1>"
  Bus Selector/2 -> Data Store Write/2  "<signal2>"
  Bus Selector/3 -> Data Store Write/3  "<Buffer_4>"
  Constant/1 -> Sum/1
  delay_estimation_1/1 -> Sum/3
  Sum/1 -> [expected_LT_CAN1], Demux message CAN1 and check coherence/2(expected_local_time)
  Constant1/1 -> Sum1/1
  expected_local_time/1 -> Sum1/2, Sum/2
  delay_estimation_2/1 -> Sum1/3
  Sum1/1 -> [expected_LT_CAN2], Demux message CAN2 and check coherence/2(expected_local_time)
  Data Store Read1/1 -> Minus/2
  Switch1/1 -> Data Store Write2/1  "Desync_Vote3_s"
  new_CAN1_msg/1 -> Switch1/2, Demux message CAN1 and check coherence/Enable
  [expected_LT_CAN2] -> Minus/1
  Data Store Read/1 -> Minus1/2
  [expected_LT_CAN1] -> Minus1/1
  Minus1/1 -> Switch1/1
  Minus/1 -> Switch1/3

== system HANcoder_E407_GTSync_v5/HANcoder STM32 Target - E407-STM32 algorithm/Global Ticks Increment/CAN Management/Matrix Cycle Manager/COMP Task - Update LT/Local Time Update ==
  note: If the desync is negative, the Local Time
      | gets updated straight away. Otherwise,
      | the Local Time must be updated in small
      | steps.
  note: Desync Check
  note: Local Time Update Acknowledge
  note: Function call Counter - DEBUG
  note: Reset New Master Flag
  note: Global - Local time update acknowledge
  note: Logic Analyzer - DEBUG
      | Start of COMP task
  note: Logic Analyzer - DEBUG
  Enable : EnablePort
  Constant : Constant  Priority=26  Value=0  OutDataTypeStr=boolean
  Constant1 : Constant  Priority=28  OutDataTypeStr=boolean
  Constant2 : Constant  Priority=31  OutDataTypeStr=int32
  Constant3 : Constant  Priority=24  OutDataTypeStr=boolean
  Constant4 : Constant  Value=0
  Data Store Read1 : DataStoreRead  Priority=11  DataStoreName=Desync_Ticks
  Data Store Read4 : DataStoreRead  Priority=30  DataStoreName=LT_Update_Counter
  Data Store Write : DataStoreWrite  DataStoreName=Desync_Positive
  Data Store Write13 : DataStoreWrite  Priority=25  DataStoreName=sync_processed
  Data Store Write2 : DataStoreWrite  Priority=27  DataStoreName=New_Master
  Data Store Write3 : DataStoreWrite  Priority=29  DataStoreName=Toggle_Pin_A0
  Data Store Write4 : DataStoreWrite  Priority=33  DataStoreName=LT_Update_Counter
  Desync_Negative : Subsystem  TreatAsAtomicUnit=on
  GreaterThan : RelationalOperator  Operator=>  OutDataTypeStr=boolean  RndMeth=Simplest
  NOT : Logic  Operator=NOT  IconShape=distinctive  AllPortsSameDT=off  OutDataTypeStr=boolean
  Plus : Sum  Priority=32
  wires:
  Constant/1 -> Data Store Write2/1
  Constant1/1 -> Data Store Write3/1
  Data Store Read4/1 -> Plus/1
  Plus/1 -> Data Store Write4/1  "LT_Update_Counter_bc0_s"
  Constant2/1 -> Plus/2
  Constant3/1 -> Data Store Write13/1
  Data Store Read1/1 -> GreaterThan/1
  Constant4/1 -> GreaterThan/2
  NOT/1 -> Desync_Negative/Enable
  GreaterThan/1 -> NOT/1, Data Store Write/1

== system HANcoder_E407_GTSync_v5/HANcoder STM32 Target - E407-STM32 algorithm/Global Ticks Increment/CAN Management/Matrix Cycle Manager/COMP Task - Update LT - bc1/Local Time Update ==
  note: Current Local Time correction
  note: Reset New Master Flag
  note: Function call Counter - DEBUG
  note: Local Time Update Acknowledge
  note: Local Time Update
  note: Global - Local time update acknowledge
  note: Logic Analyzer - DEBUG
  note: Logic Analyzer - DEBUG
      | Start of COMP task
  note: Wait until new message
      | arrives
  note: Wait until new message
      | arrives
  Enable : EnablePort
  Cast : DataTypeConversion  OutDataTypeStr=uint16
  Constant : Constant  Value=0  OutDataTypeStr=boolean
  Constant1 : Constant  OutDataTypeStr=boolean
  Constant2 : Constant  OutDataTypeStr=int32
  Constant3 : Constant  OutDataTypeStr=boolean
  Current_local_time : Constant  Value=TM_Update_LT  OutDataTypeStr=uint16
  Data Store Read : DataStoreRead  DataStoreName=Desync_Ticks
  Data Store Read4 : DataStoreRead  DataStoreName=LT_Update_Counter
  Data Store Write1 : DataStoreWrite  DataStoreName=Local_Ticks  DataStoreElements=Local_Ticks
  Data Store Write13 : DataStoreWrite  DataStoreName=sync_processed
  Data Store Write2 : DataStoreWrite  DataStoreName=New_Master
  Data Store Write3 : DataStoreWrite  DataStoreName=Toggle_Pin_A0
  Data Store Write4 : DataStoreWrite  DataStoreName=LT_Update_Counter
  Data Store Write5 : DataStoreWrite  DataStoreName=New_Msg_Ready_CAN1
  Data Store Write6 : DataStoreWrite  DataStoreName=New_Msg_Ready_CAN2
  Minus : Sum
  Plus : Sum
  RESET : Constant  Value=0  OutDataTypeStr=boolean
  RESET1 : Constant  Value=0  OutDataTypeStr=boolean
  wires:
  Current_local_time/1 -> Minus/1
  Data Store Read/1 -> Minus/2
  RESET1/1 -> Data Store Write6/1
  RESET/1 -> Data Store Write5/1
  Minus/1 -> Cast/1  "RX_LT_Master_bc1_s"
  Constant1/1 -> Data Store Write3/1
  Data Store Read4/1 -> Plus/1
  Constant3/1 -> Data Store Write13/1
  Constant2/1 -> Plus/2
  Plus/1 -> Data Store Write4/1  "LT_Update_Counter_bc1_s"
  Constant/1 -> Data Store Write2/1
  Cast/1 -> Data Store Write1/1

== system HANcoder_E407_GTSync_v5/HANcoder STM32 Target - E407-STM32 algorithm/Global Ticks Increment/CAN Management/Matrix Cycle Manager/COMP Task - Vote Decision/Vote Decision ==
  note: Vote for lowest error count (lowest id wins at tie)
  note: Logic Analyzer - DEBUG
  note: Logic Analyzer - DEBUG
      | Start of COMP task
  Enable : EnablePort
  Cast : DataTypeConversion  Priority=21  OutDataTypeStr=uint8
  Constant : Constant  Priority=6
  Constant1 : Constant  Priority=7  Value=2
  Constant2 : Constant  Priority=8  Value=3
  Constant3 : Constant  Priority=23  OutDataTypeStr=boolean
  Constant4 : Constant  Priority=15
  Constant5 : Constant  Priority=16  Value=2
  Constant6 : Constant  Priority=17  Value=3
  Data Store Read : DataStoreRead  Priority=2  DataStoreName=sync_processed
  Data Store Read1 : DataStoreRead  Priority=3  DataStoreName=Board1_error_counter
  Data Store Read2 : DataStoreRead  Priority=4  DataStoreName=Board2_error_counter
  Data Store Read21 : DataStoreRead  Priority=1  DataStoreName=Master_ID
  Data Store Read3 : DataStoreRead  Priority=5  DataStoreName=Board3_error_counter
  Data Store Write3 : DataStoreWrite  Priority=24  DataStoreName=Toggle_Pin_A0
  Data Store Write5 : DataStoreWrite  Priority=22  DataStoreName=Vote
  Ensure no self votes or failed master reelected : Subsystem  Priority=9
  Ensure no self votes or failed master reelected1 : Subsystem  Priority=10
  Ensure no self votes or failed master reelected2 : Subsystem  Priority=11
  Equal : RelationalOperator  Priority=13  Operator===  OutDataTypeStr=boolean  RndMeth=Simplest
  Equal5 : RelationalOperator  Priority=14  Operator===  OutDataTypeStr=boolean  RndMeth=Simplest
  Max : MinMax  Priority=12  Inputs=3
  Switch5 : Switch  Priority=20  Criteria=u2 > Threshold
  Switch6 : Switch  Priority=19  Criteria=u2 > Threshold
  Switch7 : Switch  Priority=18  Criteria=u2 > Threshold
  wires:
  Cast/1 -> Data Store Write5/1  "Vote_s"
  Equal/1 -> Switch6/2
  Data Store Read/1 -> Ensure no self votes or failed master reelected2/2(Sync Timeout), Ensure no self votes or failed master reelected1/2(Sync Timeout), Ensure no self votes or failed master reelected/2(Sync Timeout), Switch5/2
  Switch5/1 -> Cast/1
  Switch6/1 -> Switch5/3
  Data Store Read21/1 -> Switch5/1
  Ensure no self votes or failed master reelected2/1(Out1) -> Max/3
  Constant5/1 -> Switch7/1
  Ensure no self votes or failed master reelected1/1(Out1) -> Max/2, Equal5/2
  Constant4/1 -> Switch6/1
  Constant6/1 -> Switch7/3
  Switch7/1 -> Switch6/3
  Constant1/1 -> Ensure no self votes or failed master reelected1/1(Node ID)
  Constant2/1 -> Ensure no self votes or failed master reelected2/1(Node ID)
  Data Store Read1/1 -> Ensure no self votes or failed master reelected/3(Error counter)
  Equal5/1 -> Switch7/2
  Constant/1 -> Ensure no self votes or failed master reelected/1(Node ID)
  Max/1 -> Equal/2, Equal5/1
  Ensure no self votes or failed master reelected/1(Out1) -> Equal/1, Max/1
  Data Store Read2/1 -> Ensure no self votes or failed master reelected1/3(Error counter)
  Data Store Read3/1 -> Ensure no self votes or failed master reelected2/3(Error counter)
  Constant3/1 -> Data Store Write3/1
